simulink model "f1transferFun"  (R2024a)
settings: Solver=VariableStepAuto  StartTime=0.0  StopTime=12  RelTol=1e-3
settings Model: LastModifiedBy=użytkownik

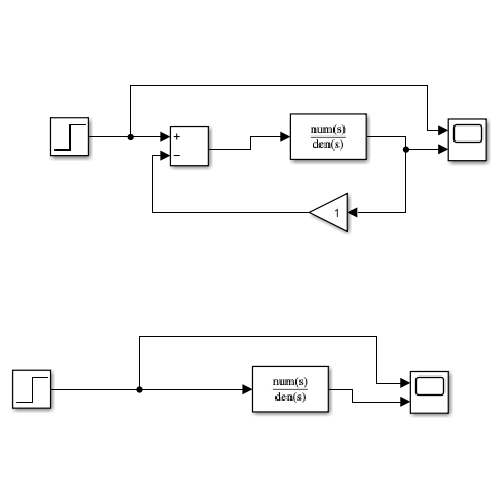
[thumbnail: Simulink's stored preview of the top-level diagram]
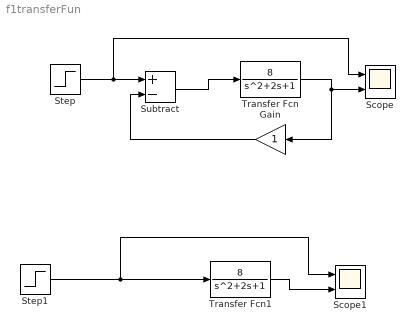
== system f1transferFun ==
  Gain : Gain
  Scope : Scope  NumInputPorts=2
  Scope1 : Scope  NumInputPorts=2
  Step : Step  After=5  SampleTime=0
  Step1 : Step  SampleTime=0
  Subtract : Sum  Inputs=+-
  Transfer Fcn : TransferFcn  Numerator=[8]
  Transfer Fcn1 : TransferFcn  Numerator=[8]
  wires:
  Transfer Fcn1/1 -> Scope1/2
  Gain/1 -> Subtract/2
  Transfer Fcn/1 -> Gain/1, Scope/2
  Subtract/1 -> Transfer Fcn/1
  Step/1 -> Scope/1, Subtract/1
  Step1/1 -> Scope1/1, Transfer Fcn1/1
